simulink model "TST_InjCrv_MI1SOEAirMsCor"  (R2016b)
settings: Solver=FixedStepDiscrete  StartTime=0.0  StopTime=5  FixedStep=1  RelTol=1e-3
settings Model: Creator=WF305  LastModifiedBy=WF305
settings DebuggingCC: SignalRangeChecking=error

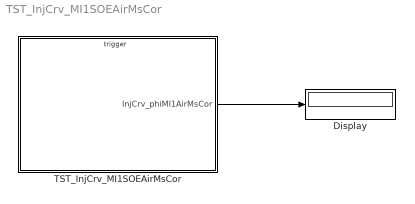
== system TST_InjCrv_MI1SOEAirMsCor ==
  Display : Display
  TST_InjCrv_MI1SOEAirMsCor : Subsystem
  wires:
  TST_InjCrv_MI1SOEAirMsCor/1(InjCrv_phiMI1AirMsCor) -> Display/1

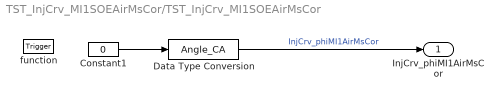
== system TST_InjCrv_MI1SOEAirMsCor/TST_InjCrv_MI1SOEAirMsCor ==
  function : TriggerPort  TriggerType=function-call  VariantControl=Variant
  Constant1 : Constant  Value=0
  Data Type Conversion : DataTypeConversion  OutDataTypeStr=Angle_CA
  InjCrv_phiMI1AirMsCor : Outport  Tag=CA  Description=The dynamic correction value is calculated as the compensation based on the air quality deviation  OutMin=-10  OutMax=40  OutDataTypeStr=Angle_CA
  wires:
  Constant1/1 -> Data Type Conversion/1
  Data Type Conversion/1 -> InjCrv_phiMI1AirMsCor/1  "InjCrv_phiMI1AirMsCor"
